simulink model "control_system_sim"  (R2017b)
settings: Solver=VariableStepAuto  StartTime=0.0  StopTime=tmax  RelTol=1e-3
undefined symbols (not defined in the file): Beq, F_load, f_pwm, Im_max, Jeq, Kdp, Kdv, Kip, Kiv, Km, Kpp, Kpv, Kt, Lm, Rm, ts, Vin_pwm, Vout_pwm
libraries: simulink x4
settings Model: Creator=JesusC  LastModifiedBy=JesusC

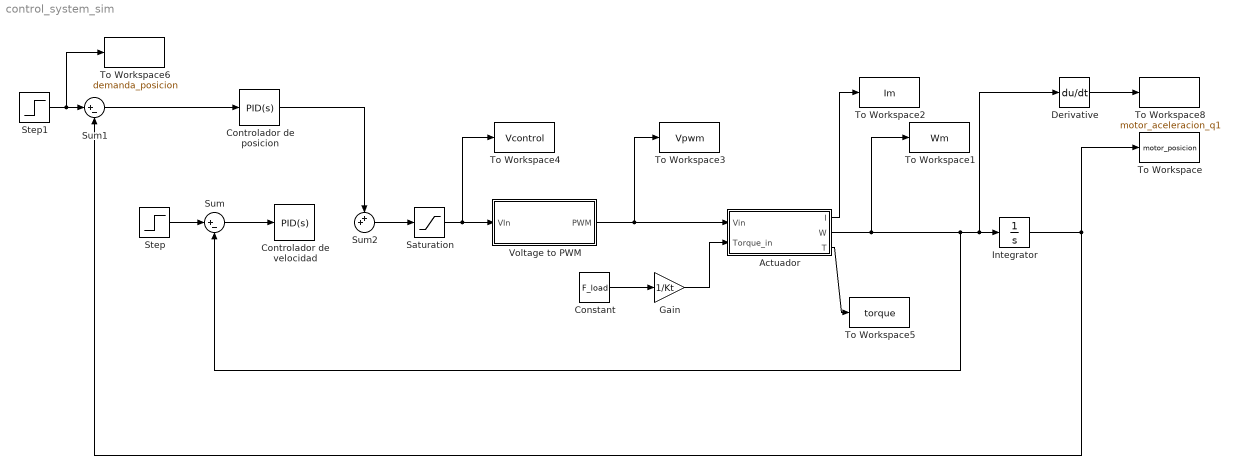
== system control_system_sim ==
  "Actuador " : Subsystem
  Constant : Constant  Value=F_load  VectorParams1D=off  SampleTime=ts
  Controlador de posicion : simulink/Continuous/PID Controller  Controller=PID  TimeDomain=Continuous-time  SampleTime=-1  IntegratorMethod=Forward Euler  FilterMethod=Forward Euler  Form=Parallel  UseFilter=on  ControllerParametersSource=internal  P=Kpp  I=Kip  D=Kdp  N=10000  InitialConditionSource=internal  InitialConditionForIntegrator=0  InitialConditionForFilter=0  ExternalReset=none  LimitOutput=off  UpperSaturationLimit=inf  LowerSaturationLimit=-inf  LinearizeAsGain=on  AntiWindupMode=none  Kb=1  TrackingMode=off  Kt=1  PParamMin=[]  PParamMax=[]  IParamMin=[]  IParamMax=[]  DParamMin=[]  DParamMax=[]  NParamMin=[]  NParamMax=[]  KbParamMin=[]  KbParamMax=[]  KtParamMin=[]  KtParamMax=[]  POutMin=[]  POutMax=[]  IOutMin=[]  IOutMax=[]  DOutMin=[]  DOutMax=[]  NOutMin=[]  NOutMax=[]  KbOutMin=[]  KbOutMax=[]  KtOutMin=[]  KtOutMax=[]  IntegratorOutMin=[]  IntegratorOutMax=[]  FilterOutMin=[]  FilterOutMax=[]  SumOutMin=[]  SumOutMax=[]  SumI1OutMin=[]  SumI1OutMax=[]  SumI2OutMin=[]  SumI2OutMax=[]  SumI3OutMin=[]  SumI3OutMax=[]  SumDOutMin=[]  SumDOutMax=[]  SaturationOutMin=[]  SaturationOutMax=[]  IntegratorContinuousStateAttributes=''  IntegratorStateMustResolveToSignalObject=off  IntegratorRTWStateStorageClass=Auto  FilterContinuousStateAttributes=''  FilterStateMustResolveToSignalObject=off  FilterRTWStateStorageClass=Auto  DifferentiatorICPrevScaledInput=0  DifferentiatorOutMin=[]  DifferentiatorOutMax=[]  InitialConditionSetting=State (most efficient)  FilterDiffOutCoefMin=[]  FilterDiffOutCoefMax=[]  SumDenOutMin=[]  SumDenOutMax=[]  SumNumOutMin=[]  SumNumOutMax=[]  ReciprocalOutMin=[]  ReciprocalOutMax=[]  DivideOutMin=[]  DivideOutMax=[]  TunerSelectOption=Transfer Function Based (PID Tuner App)
  Controlador de velocidad : simulink/Continuous/PID Controller  Controller=PID  TimeDomain=Continuous-time  SampleTime=-1  IntegratorMethod=Forward Euler  FilterMethod=Forward Euler  Form=Parallel  UseFilter=on  ControllerParametersSource=internal  P=Kpv  I=Kiv  D=Kdv  N=10000  InitialConditionSource=internal  InitialConditionForIntegrator=0  InitialConditionForFilter=0  ExternalReset=none  LimitOutput=off  UpperSaturationLimit=inf  LowerSaturationLimit=-inf  LinearizeAsGain=on  AntiWindupMode=none  Kb=1  TrackingMode=off  Kt=1  PParamMin=[]  PParamMax=[]  IParamMin=[]  IParamMax=[]  DParamMin=[]  DParamMax=[]  NParamMin=[]  NParamMax=[]  KbParamMin=[]  KbParamMax=[]  KtParamMin=[]  KtParamMax=[]  POutMin=[]  POutMax=[]  IOutMin=[]  IOutMax=[]  DOutMin=[]  DOutMax=[]  NOutMin=[]  NOutMax=[]  KbOutMin=[]  KbOutMax=[]  KtOutMin=[]  KtOutMax=[]  IntegratorOutMin=[]  IntegratorOutMax=[]  FilterOutMin=[]  FilterOutMax=[]  SumOutMin=[]  SumOutMax=[]  SumI1OutMin=[]  SumI1OutMax=[]  SumI2OutMin=[]  SumI2OutMax=[]  SumI3OutMin=[]  SumI3OutMax=[]  SumDOutMin=[]  SumDOutMax=[]  SaturationOutMin=[]  SaturationOutMax=[]  IntegratorContinuousStateAttributes=''  IntegratorStateMustResolveToSignalObject=off  IntegratorRTWStateStorageClass=Auto  FilterContinuousStateAttributes=''  FilterStateMustResolveToSignalObject=off  FilterRTWStateStorageClass=Auto  DifferentiatorICPrevScaledInput=0  DifferentiatorOutMin=[]  DifferentiatorOutMax=[]  InitialConditionSetting=State (most efficient)  FilterDiffOutCoefMin=[]  FilterDiffOutCoefMax=[]  SumDenOutMin=[]  SumDenOutMax=[]  SumNumOutMin=[]  SumNumOutMax=[]  ReciprocalOutMin=[]  ReciprocalOutMax=[]  DivideOutMin=[]  DivideOutMax=[]  TunerSelectOption=Transfer Function Based (PID Tuner App)
  Derivative : Derivative  CoefficientInTFapproximation=0
  Gain : Gain  Gain=1/Kt
  Integrator : Integrator
  Saturation : Saturate  UpperLimit=Vin_pwm  LowerLimit=-Vin_pwm
  Step : Step  Time=2  Before=100  After=105  SampleTime=0
  Step1 : Step  Before=100  After=105  SampleTime=0
  Sum : Sum  Inputs=|+-
  Sum1 : Sum  Inputs=|+-
  Sum2 : Sum  Inputs=++|
  To Workspace : ToWorkspace  VariableName=motor_posicion  SampleTime=ts
      settings: MaxDataPoints=N
  To Workspace1 : ToWorkspace  VariableName=Wm  SampleTime=ts
      settings: MaxDataPoints=N
  To Workspace2 : ToWorkspace  VariableName=Im  SampleTime=ts
      settings: MaxDataPoints=N
  To Workspace3 : ToWorkspace  VariableName=Vpwm  SampleTime=ts
      settings: MaxDataPoints=N
  To Workspace4 : ToWorkspace  VariableName=Vcontrol  SampleTime=ts
      settings: MaxDataPoints=N
  To Workspace5 : ToWorkspace  VariableName=torque  SampleTime=ts
      settings: MaxDataPoints=N
  To Workspace6 : ToWorkspace  VariableName=demanda_posicion  SampleTime=ts
      settings: MaxDataPoints=N
  To Workspace8 : ToWorkspace  VariableName=motor_aceleracion_q1  SampleTime=ts
      settings: MaxDataPoints=N
  Voltage to PWM : Subsystem
  wires:
  Step/1 -> Sum/1
  Sum/1 -> Controlador de velocidad/1
  Integrator/1 -> Sum1/2, To Workspace/1
  Saturation/1 -> To Workspace4/1, Voltage to PWM/1(VIn)
  Gain/1 -> "Actuador "/2(Torque_in)
  Derivative/1 -> To Workspace8/1
  "Actuador "/1(I) -> To Workspace2/1
  "Actuador "/2(W) -> To Workspace1/1, Sum/2, Derivative/1, Integrator/1
  "Actuador "/3(T) -> To Workspace5/1
  Voltage to PWM/1(PWM) -> To Workspace3/1, "Actuador "/1(Vin)
  Constant/1 -> Gain/1
  Sum2/1 -> Saturation/1
  Sum1/1 -> Controlador de posicion/1
  Step1/1 -> To Workspace6/1, Sum1/1
  Controlador de posicion/1 -> Sum2/1

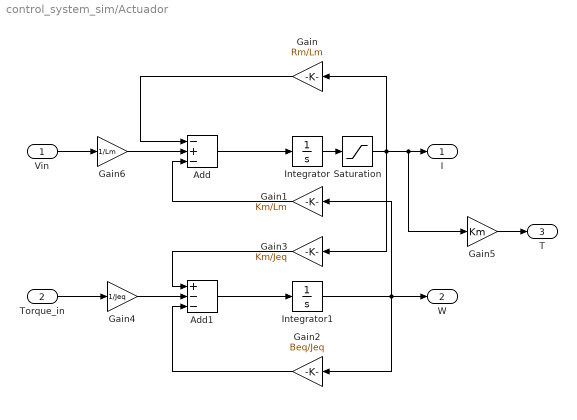
== system control_system_sim/Actuador  ==
  Vin : Inport
  Torque_in : Inport  Port=2
  Add : Sum  Inputs=-+-
  Add1 : Sum  Inputs=+--
  Gain : Gain  Gain=Rm/Lm
  Gain1 : Gain  Gain=Km/Lm
  Gain2 : Gain  Gain=Beq/Jeq
  Gain3 : Gain  Gain=Km/Jeq
  Gain4 : Gain  Gain=1/Jeq
  Gain5 : Gain  Gain=Km
  Gain6 : Gain  Gain=1/Lm
  Integrator : Integrator
  Integrator1 : Integrator
  Saturation : Saturate  UpperLimit=Im_max  LowerLimit=-Im_max
  I : Outport
  W : Outport  Port=2
  T : Outport  Port=3
  wires:
  Integrator/1 -> Saturation/1
  Gain/1 -> Add/1
  Integrator1/1 -> Gain2/1, Gain1/1, W/1
  Gain1/1 -> Add/3
  Add/1 -> Integrator/1
  Add1/1 -> Integrator1/1
  Gain2/1 -> Add1/3
  Gain3/1 -> Add1/1
  Torque_in/1 -> Gain4/1
  Gain4/1 -> Add1/2
  Gain5/1 -> T/1
  Vin/1 -> Gain6/1
  Gain6/1 -> Add/2
  Saturation/1 -> Gain3/1, Gain/1, Gain5/1, I/1

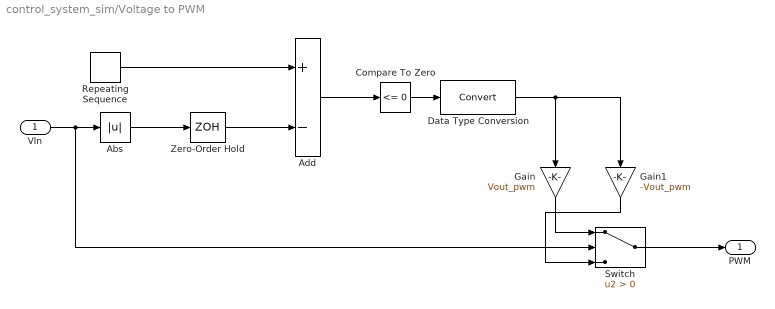
== system control_system_sim/Voltage to PWM ==
  VIn : Inport
  Abs : Abs
  Add : Sum  Inputs=+-
  Compare To Zero : simulink/Logic and Bit Operations/Compare To Zero  relop=<=  OutDataTypeStr=boolean
  Data Type Conversion : DataTypeConversion
  Gain : Gain  Gain=Vout_pwm
  Gain1 : Gain  Gain=-Vout_pwm
  Repeating Sequence : simulink/Sources/Repeating Sequence  rep_seq_t=[0 1/f_pwm]  rep_seq_y=[0 Vin_pwm]
  Switch : Switch  Criteria=u2 > Threshold
  Zero-Order Hold : ZeroOrderHold  SampleTime=-1
  PWM : Outport
  wires:
  Repeating Sequence/1 -> Add/1
  Add/1 -> Compare To Zero/1
  Zero-Order Hold/1 -> Add/2
  Abs/1 -> Zero-Order Hold/1
  VIn/1 -> Switch/2, Abs/1
  Gain/1 -> Switch/1
  Gain1/1 -> Switch/3
  Compare To Zero/1 -> Data Type Conversion/1
  Switch/1 -> PWM/1
  Data Type Conversion/1 -> Gain/1, Gain1/1
